simulink model "ACC"  (R2020a)
settings: Solver=FixedStepAuto  StartTime=0.0  StopTime=200  RelTol=1e-3  EnableMultiTasking=on
undefined symbols (not defined in the file): gray
libraries: embdlinuxlib x5, simulink x2, raspberrypiBasiclib x2, dspmtrx3 x1, visionanalysis x1, fuzblock x1, visiongeotforms x1, visiontextngfix x1
settings Model: SimulationMode=external  Creator=Administrator  LastModifiedBy=zhengliang
settings SolverCC: PositivePriorityOrder=on  AutoInsertRateTranBlk=on
settings DataIOCC: ReturnWorkspaceOutputs=off
settings OptimizationCC: EnhancedBackFolding=on  PassReuseOutputArgsAs=Individual arguments  MaxStackSize=64  OptimizeBlockOrder=speed  DifferentSizesBufferReuse=on  OptimizationCustomize=off  EfficientTunableParamExpr=on
settings DebuggingCC: ParameterTunabilityLossMsg=error  ArithmeticOperatorsInVariantConditions=warning
settings HardwareCC: ProdBitPerPointer=32  ProdBitPerSizeT=32  ProdBitPerPtrDiffT=32  ProdLargestAtomicInteger=Long  ProdLargestAtomicFloat=Double  ProdWordSize=32  ProdHWDeviceType=ARM Compatible->ARM Cortex
settings SFSimCC: MATLABDynamicMemAlloc=off  CustomCodeUndefinedFunction=UseInterfaceOnly
settings RTWCC: SystemTargetFile=ert.tlc  HardwareBoard=Raspberry Pi  TemplateMakefile=ert_default_tmf  GenerateReport=on  Toolchain=GNU GCC Raspberry Pi  BuildConfiguration=Faster Runs  IncludeHyperlinkInReport=on  LaunchReport=on  GenerateTraceInfo=on  GenerateTraceReport=on  GenerateTraceReportSl=on  GenerateTraceReportSf=on  GenerateTraceReportEml=on
settings CodeAppCC: ForceParamTrailComments=on  IgnoreCustomStorageClasses=off  OperatorAnnotations=on  SimulinkDataObjDesc=on  SFDataObjDesc=on  InsertBlockDesc=on
settings ERTTargetCC: SupportContinuousTime=on  SupportVariableSizeSignals=on

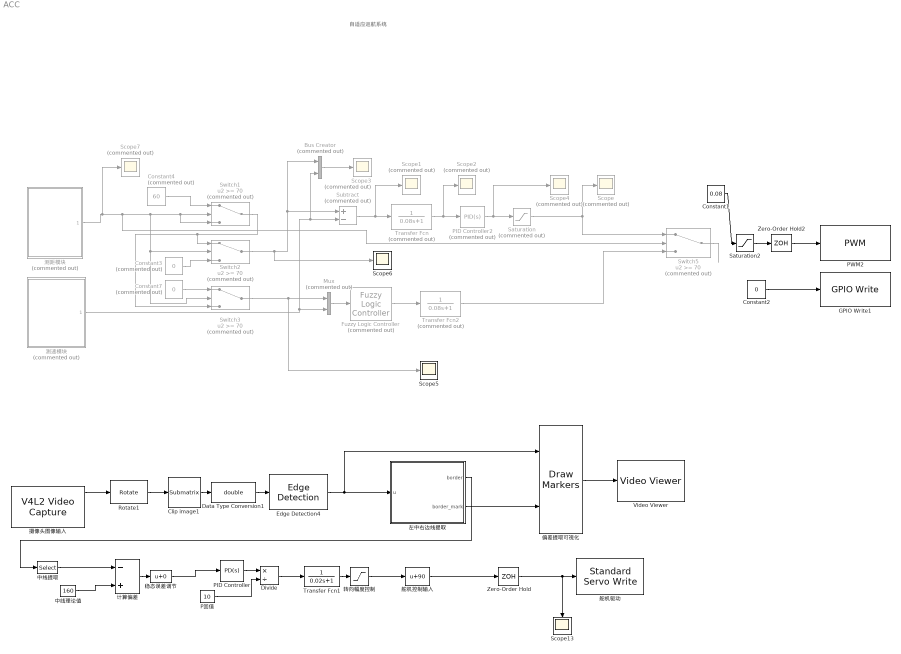
== system ACC ==
  note: 自适应巡航系统
  Bus Creator : BusCreator  Commented=on  Inputs=2
  Clip image1 : dspmtrx3/Submatrix  RowSpan=Range of rows  RowStartMode=Index  RowStartIndex=100  RowEndMode=Index  RowEndIndex=200  ColSpan=All columns  ColStartMode=First  ColStartIndex=1  ColEndMode=Last  ColEndIndex=1
  Constant1 : Constant  Value=0.08
  Constant2 : Constant  Value=0
  Constant3 : Constant  Commented=on  Value=0
  Constant4 : Constant  Commented=on  Value=60
  Constant7 : Constant  Commented=on  Value=0
  Data Type Conversion1 : DataTypeConversion  OutDataTypeStr=double
  Divide : Product  Inputs=*/
  Edge Detection4 : visionanalysis/Edge Detection  method=Sobel  outputType=Binary image  userDefinedThreshold=on  thresholdSource=Specify via dialog  threshold=22  thresholdTuning=1  edgeThinning=on  threshold_canny=[0.25 0.60]  autoPercent=90  sigma=1  roundingMode=Floor  overflowMode=off  prodOutputMode=Binary point scaling  prodOutputWordLength=32  prodOutputFracLength=8
      settings: SourceProductBaseCode=VP
  Fuzzy Logic Controller : fuzblock/Fuzzy Logic  Controller  Commented=on  FIS='tipper.fis'  OutputSampleNumber=101  DataType=double  FuzzifiedInputs=off  RuleFiringStrengths=off  RuleOutputs=off  AggregatedOutputs=off  SimulateUsing=Interpreted execution  OutOfRangeInputValueMessage=warning  NoRuleFiredMessage=warning  EmptyOutputFuzzySetMessage=warning
  GPIO Write1 : embdlinuxlib/GPIO Write  board=Pi 3 Model B+  gpio=27  direction=Output  blockPlatform=Raspberry Pi
      settings: SourceProductBaseCode=SC_BEAGLEBONE_BLUE,RASPPI
  Mux : Mux  Commented=on  Inputs=2
  PID Controller : simulink/Continuous/PID Controller  Controller=PD  Form=Parallel  TimeDomain=Continuous-time  UseExternalTs=off  SampleTime=-1  IntegratorMethod=Forward Euler  FilterMethod=Forward Euler  ControllerParametersSource=internal  P=15  I=0.001  D=0.8  UseFilter=on  N=3  TunerSelectOption=Transfer Function Based (PID Tuner App)  InitialConditionSource=internal  InitialConditionForIntegrator=0  InitialConditionForFilter=0  DifferentiatorICPrevScaledInput=0  ExternalReset=none  TrackingMode=off  Kt=1  LimitOutput=off  UpperSaturationLimit=inf  LowerSaturationLimit=-inf  LinearizeAsGain=on  AntiWindupMode=none  Kb=1  POutMin=[]  POutMax=[]  IOutMin=[]  IOutMax=[]  DOutMin=[]  DOutMax=[]  NOutMin=[]  NOutMax=[]  SumOutMin=[]  SumOutMax=[]  SaturationOutMin=[]  SaturationOutMax=[]  PParamMin=[]  PParamMax=[]  IParamMin=[]  IParamMax=[]  DParamMin=[]  DParamMax=[]  NParamMin=[]  NParamMax=[]  KbParamMin=[]  KbParamMax=[]  KtParamMin=[]  KtParamMax=[]  KbOutMin=[]  KbOutMax=[]  KtOutMin=[]  KtOutMax=[]  IntegratorOutMin=[]  IntegratorOutMax=[]  FilterOutMin=[]  FilterOutMax=[]  SumI1OutMin=[]  SumI1OutMax=[]  SumI2OutMin=[]  SumI2OutMax=[]  SumI3OutMin=[]  SumI3OutMax=[]  SumI4OutMin=[]  SumI4OutMax=[]  SumDOutMin=[]  SumDOutMax=[]  DifferentiatorOutMin=[]  DifferentiatorOutMax=[]  FilterDiffOutCoefMin=[]  FilterDiffOutCoefMax=[]  ReciprocalOutMin=[]  ReciprocalOutMax=[]  SumDenOutMin=[]  SumDenOutMax=[]  SumNumOutMin=[]  SumNumOutMax=[]  DivideOutMin=[]  DivideOutMax=[]  UdiffTsProdOutMin=[]  UdiffTsProdOutMax=[]  NTsProdOutMin=[]  NTsProdOutMax=[]  UintegralTsProdOutMin=[]  UintegralTsProdOutMax=[]  UngainTsProdOutMin=[]  UngainTsProdOutMax=[]  IntegratorContinuousStateAttributes=''  IntegratorStateMustResolveToSignalObject=off  IntegratorRTWStateStorageClass=Auto  FilterContinuousStateAttributes=''  FilterStateMustResolveToSignalObject=off  FilterRTWStateStorageClass=Auto  ParallelPVariant=InternalParameters  IdealPVariant=Disabled  IVariant=Disabled  DVariant=InternalParameters  IntegratorVariant=Disabled  SatVariant=Disabled  AWVariant=Disabled  PCopyVariant=Disabled  TRVariant=Disabled  FdbkBlocksVariant=Forward  IdealPFdbkVariant=Disabled  SatFdbkVariant=Disabled  DerivativeFilterVariant=ContFilter  NVariant=InternalParameters  NCopyVariant=Disabled  FilterICVariant=InternalICsFilter  IntegratorICVariant=Disabled  ExternalResetVariant=Disabled  TRSumVariant=Passthrough  SumFdbkVariant=Disabled  SumVariant=Sum_PD  TsampFilterVariant=InternalTs  TsampNgainVariant=Passthrough  TsampIntegralVariant=Disabled_SignalSpec
  PID Controller2 : simulink/Continuous/PID Controller  Commented=on  Controller=PID  Form=Parallel  TimeDomain=Continuous-time  UseExternalTs=off  SampleTime=-1  IntegratorMethod=Forward Euler  FilterMethod=Forward Euler  ControllerParametersSource=internal  P=0.001  I=0.00005  D=0  UseFilter=on  N=100  TunerSelectOption=Transfer Function Based (PID Tuner App)  InitialConditionSource=internal  InitialConditionForIntegrator=0  InitialConditionForFilter=0  DifferentiatorICPrevScaledInput=0  ExternalReset=none  TrackingMode=off  Kt=1  LimitOutput=off  UpperSaturationLimit=inf  LowerSaturationLimit=-inf  LinearizeAsGain=on  AntiWindupMode=none  Kb=1  POutMin=[]  POutMax=[]  IOutMin=[]  IOutMax=[]  DOutMin=[]  DOutMax=[]  NOutMin=[]  NOutMax=[]  SumOutMin=[]  SumOutMax=[]  SaturationOutMin=[]  SaturationOutMax=[]  PParamMin=[]  PParamMax=[]  IParamMin=[]  IParamMax=[]  DParamMin=[]  DParamMax=[]  NParamMin=[]  NParamMax=[]  KbParamMin=[]  KbParamMax=[]  KtParamMin=[]  KtParamMax=[]  KbOutMin=[]  KbOutMax=[]  KtOutMin=[]  KtOutMax=[]  IntegratorOutMin=[]  IntegratorOutMax=[]  FilterOutMin=[]  FilterOutMax=[]  SumI1OutMin=[]  SumI1OutMax=[]  SumI2OutMin=[]  SumI2OutMax=[]  SumI3OutMin=[]  SumI3OutMax=[]  SumI4OutMin=[]  SumI4OutMax=[]  SumDOutMin=[]  SumDOutMax=[]  DifferentiatorOutMin=[]  DifferentiatorOutMax=[]  FilterDiffOutCoefMin=[]  FilterDiffOutCoefMax=[]  ReciprocalOutMin=[]  ReciprocalOutMax=[]  SumDenOutMin=[]  SumDenOutMax=[]  SumNumOutMin=[]  SumNumOutMax=[]  DivideOutMin=[]  DivideOutMax=[]  UdiffTsProdOutMin=[]  UdiffTsProdOutMax=[]  NTsProdOutMin=[]  NTsProdOutMax=[]  UintegralTsProdOutMin=[]  UintegralTsProdOutMax=[]  UngainTsProdOutMin=[]  UngainTsProdOutMax=[]  IntegratorContinuousStateAttributes=''  IntegratorStateMustResolveToSignalObject=off  IntegratorRTWStateStorageClass=Auto  FilterContinuousStateAttributes=''  FilterStateMustResolveToSignalObject=off  FilterRTWStateStorageClass=Auto  ParallelPVariant=InternalParameters  IdealPVariant=Disabled  IVariant=InternalParameters  DVariant=InternalParameters  IntegratorVariant=Continuous  SatVariant=Disabled  AWVariant=Passthrough  PCopyVariant=Disabled  TRVariant=Disabled  FdbkBlocksVariant=Forward  IdealPFdbkVariant=Disabled  SatFdbkVariant=Disabled  DerivativeFilterVariant=ContFilter  NVariant=InternalParameters  NCopyVariant=Disabled  FilterICVariant=InternalICsFilter  IntegratorICVariant=InternalICs  ExternalResetVariant=Disabled  TRSumVariant=Passthrough  SumFdbkVariant=Disabled  SumVariant=Sum_PID  TsampFilterVariant=InternalTs  TsampNgainVariant=Passthrough  TsampIntegralVariant=Passthrough
  PWM2 : raspberrypiBasiclib/PWM  board=Pi 3 Model B+  Pin_=17  Frequency=8000  blockPlatform=Raspberry Pi
      settings: SourceProductBaseCode=RASPPI
  P回值 : Constant  Value=10
  Rotate1 : visiongeotforms/Rotate  outSizeR=Expanded to fit rotated input image  src_angle=Specify via dialog  unit_angle=Degrees  angle=-pi/2  maxAngle=pi  dispImage=Top-left corner  method=Table lookup  fillVal=0  interpMethod=Bilinear  roundingMode=Nearest  overflowMode=on  prodOutputMode=Binary point scaling  prodOutputWordLength=32  prodOutputFracLength=10
      settings: LockScale=on
  Saturation : Saturate  Commented=on  UpperLimit=0.071  LowerLimit=0.07
  Saturation2 : Saturate  UpperLimit=0.2  LowerLimit=0
  Scope{,1..4,7} (6 alike) : Scope  Commented=on
  Scope13 : Scope
  Scope5 : Scope
  Scope6 : Scope
  Subtract : Sum  Commented=on  Inputs=+-
  Switch{1..3,5} (4 alike) : Switch  Commented=on  Threshold=70
  Transfer Fcn : TransferFcn  Commented=on  Denominator=[0.08 1]
  Transfer Fcn1 : TransferFcn  Denominator=[0.02 1]
  Transfer Fcn2 : TransferFcn  Commented=on  Denominator=[0.08 1]
  Video Viewer : VideoViewer  colormapValue=gray(256)  FigPos=[253 673 766 511]
  Zero-Order Hold : ZeroOrderHold  SampleTime=0.05
  Zero-Order Hold2 : ZeroOrderHold  SampleTime=0.05
  中线提取 : Selector  NumberOfDimensions=2  InputPortWidth=3  IndexOptions=Index vector (dialog),Index vector (dialog)  Indices=[2],2  OutputSizes=1,1
  中线理论值 : Constant  Value=160
  偏差提取可视化 : visiontextngfix/Draw Markers  shape=Circle  size=3  fill=off  fillClrSource=Specify via dialog  display=White  intensity=200  color=[200 255 100]  opacity=0.6  viewport=Entire image  antialiasing=off  inType=Obsolete  imagePorts=One multidimensional signal  roundingMode=Floor  overflowMode=off  memoryMode=Specify word length  memoryWordLength=16  memoryFracLength=15  prodOutputMode=Binary point scaling  prodOutputWordLength=32  prodOutputFracLength=14
      settings: SourceProductBaseCode=VP
  左中右边线提取 : MATLAB Function  TreatAsAtomicUnit=on
  摄像头图像输入 : embdlinuxlib/V4L2 Video Capture  m_devName='/dev/video0'  roi=[0, 0, 640, 480]  imSizeSelection=320x240  imSize=[640, 480]  pixelFormat=RGB  pixelOrder=Planar  sampleTime=1/50  simOutput=Colorbars  blockPlatform=Raspberry Pi
      settings: SourceProductBaseCode=SC_BEAGLEBONE_BLUE,RASPPI
  "测距模块 " : Subsystem  Commented=on
  "测速模块 " : Subsystem  Commented=on
  稳态误差调节 : Bias
  舵机控制输入 : Bias  Bias=90
  舵机驱动 : raspberrypiBasiclib/Standard Servo Write  board=Pi 3 Model B+  Pin_=21  MinPulseDuration=0.96e-3  MaxPulseDuration=1.96e-3  blockPlatform=Raspberry Pi
      settings: SourceProductBaseCode=RASPPI
  计算偏差 : Sum  Inputs=-+
  转向幅度控制 : Saturate  UpperLimit=85  LowerLimit=-85
  wires:
  P回值/1 -> Divide/2
  Transfer Fcn1/1 -> 转向幅度控制/1
  Divide/1 -> Transfer Fcn1/1
  左中右边线提取/1(border) -> 中线提取/1
  Zero-Order Hold/1 -> 舵机驱动/1, Scope13/1
  舵机控制输入/1 -> Zero-Order Hold/1
  中线理论值/1 -> 计算偏差/2
  左中右边线提取/2(border_mark) -> 偏差提取可视化/2
  Clip image1/1 -> Data Type Conversion1/1
  Rotate1/1 -> Clip image1/1
  转向幅度控制/1 -> 舵机控制输入/1
  偏差提取可视化/1 -> Video Viewer/1
  稳态误差调节/1 -> PID Controller/1
  PID Controller/1 -> Divide/1
  Data Type Conversion1/1 -> Edge Detection4/1
  中线提取/1 -> 计算偏差/1
  摄像头图像输入/1 -> Rotate1/1
  计算偏差/1 -> 稳态误差调节/1
  Edge Detection4/1 -> 偏差提取可视化/1, 左中右边线提取/1(u)
  "测距模块 "/1(" ") -> Scope7/1, Switch5/2, Switch3/2, Switch2/2, Switch1/2, Switch1/3
  Constant2/1 -> GPIO Write1/1
  Saturation2/1 -> Zero-Order Hold2/1
  Zero-Order Hold2/1 -> PWM2/1
  Constant4/1 -> Switch1/1
  Saturation/1 -> Switch5/1, Scope/1
  Subtract/1 -> Scope1/1, Transfer Fcn/1
  PID Controller2/1 -> Saturation/1, Scope4/1
  Bus Creator/1 -> Scope3/1
  Transfer Fcn/1 -> PID Controller2/1, Scope2/1
  Switch1/1 -> Switch2/1, Switch3/3
  Constant3/1 -> Switch2/3
  Switch2/1 -> Scope6/1, Subtract/1, Bus Creator/1
  Constant7/1 -> Switch3/1
  Fuzzy Logic Controller/1 -> Transfer Fcn2/1
  "测速模块 "/1(" ") -> Mux/2, Subtract/2, Bus Creator/2
  Switch3/1 -> Scope5/1, Mux/1
  Mux/1 -> Fuzzy Logic Controller/1
  Transfer Fcn2/1 -> Switch5/3
  Switch5/1 -> ?
  Constant1/1 -> Saturation2/1

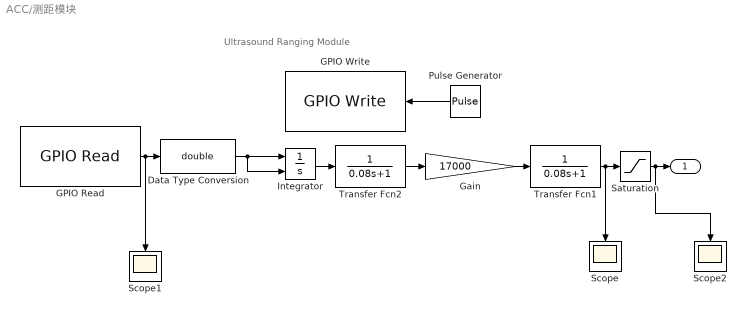
== system ACC/测距模块  ==
  note: Ultrasound Ranging Module
  Data Type Conversion : DataTypeConversion  OutDataTypeStr=double
  GPIO Read : embdlinuxlib/GPIO Read  board=Pi 3 Model B+  gpio=24  internalResistor=Off  sampleTime=inf  direction=Input  blockPlatform=Raspberry Pi
      settings: SourceProductBaseCode=SC_BEAGLEBONE_BLUE,RASPPI
  GPIO Write : embdlinuxlib/GPIO Write  board=Pi 3 Model B+  gpio=23  direction=Output  blockPlatform=Raspberry Pi
      settings: SourceProductBaseCode=SC_BEAGLEBONE_BLUE,RASPPI
  Gain : Gain  Gain=17000
  Integrator : Integrator  ExternalReset=rising
  Pulse Generator : DiscretePulseGenerator  PulseType=Time based  Period=0.1  PulseWidth=50
  Saturation : Saturate  UpperLimit=100  LowerLimit=0
  Scope : Scope
  Scope1 : Scope
  Scope2 : Scope
  Transfer Fcn1 : TransferFcn  Denominator=[0.08 1]
  Transfer Fcn2 : TransferFcn  Denominator=[0.08 1]
  " " : Outport  VectorParamsAs1DForOutWhenUnconnected=off
  wires:
  Data Type Conversion/1 -> Integrator/2, Integrator/1
  Pulse Generator/1 -> GPIO Write/1
  GPIO Read/1 -> Scope1/1, Data Type Conversion/1
  Gain/1 -> Transfer Fcn1/1
  Integrator/1 -> Transfer Fcn2/1
  Transfer Fcn1/1 -> Scope/1, Saturation/1
  Transfer Fcn2/1 -> Gain/1
  Saturation/1 -> Scope2/1, " "/1

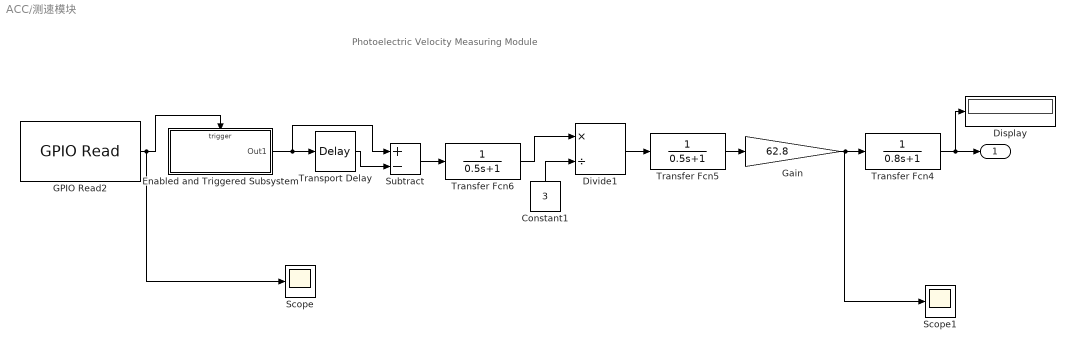
== system ACC/测速模块  ==
  note: Photoelectric Velocity Measuring Module
  Constant1 : Constant  Value=3
  Display : Display
  Divide1 : Product  Inputs=*/
  Enabled and Triggered Subsystem : Subsystem  TreatAsAtomicUnit=on
  GPIO Read2 : embdlinuxlib/GPIO Read  board=Pi 3 Model B+  gpio=21  internalResistor=Off  sampleTime=0.01  direction=Input  blockPlatform=Raspberry Pi
      settings: SourceProductBaseCode=SC_BEAGLEBONE_BLUE,RASPPI
  Gain : Gain  Gain=62.8
  Scope : Scope
  Scope1 : Scope
  Subtract : Sum  Inputs=+-
  Transfer Fcn4 : TransferFcn  Denominator=[0.8 1]
  Transfer Fcn5 : TransferFcn  Denominator=[0.5 1]
  Transfer Fcn6 : TransferFcn  Denominator=[0.5 1]
  Transport Delay : TransportDelay  DelayTime=0.5
  " " : Outport  VectorParamsAs1DForOutWhenUnconnected=off
  wires:
  Constant1/1 -> Divide1/2
  Enabled and Triggered Subsystem/1(Out1) -> Transport Delay/1, Subtract/1
  Transfer Fcn6/1 -> Divide1/1
  Transport Delay/1 -> Subtract/2
  Transfer Fcn5/1 -> Gain/1
  Divide1/1 -> Transfer Fcn5/1
  Transfer Fcn4/1 -> " "/1, Display/1
  Gain/1 -> Scope1/1, Transfer Fcn4/1
  Subtract/1 -> Transfer Fcn6/1
  GPIO Read2/1 -> Scope/1, Enabled and Triggered Subsystem/Trigger

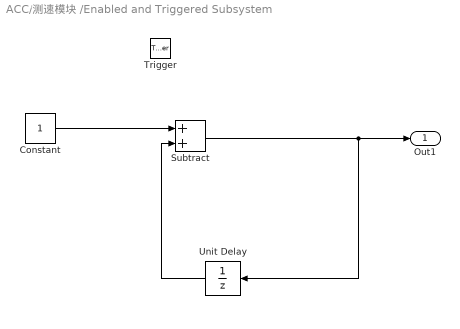
== system ACC/测速模块 /Enabled and Triggered Subsystem ==
  Trigger : TriggerPort  TriggerType=falling  VariantControl=Variant
  Constant : Constant
  Subtract : Sum
  Unit Delay : UnitDelay  SampleTime=-1  HasFrameUpgradeWarning=on
  Out1 : Outport  VectorParamsAs1DForOutWhenUnconnected=off
  wires:
  Constant/1 -> Subtract/1
  Subtract/1 -> Unit Delay/1, Out1/1
  Unit Delay/1 -> Subtract/2

== matlab function ACC/左中右边线提取 ==
  data: u input; border output; border_mark output
function [border,border_mark]= fcn(u)
scan_line=[100 75 50 25];
scan_lines=length(scan_line);
border=zeros(scan_lines,3);
[~,x_max]=size(u);
x_max_2 = x_max/2;
for i=1:scan_lines
    border(i,3)= x_max;
    border(i,2)= x_max_2;
end
mid = x_max_2;
%start to scan the border
for y=1:scan_lines
    for x_left=1:mid
        if u(scan_line(y),mid-x_left+1)==1
           border(y,1)=x_max_2-x_left;
           break
        end
    end
    for x_right=1:(x_max-mid)
        if u(scan_line(y),mid+x_right-1)==1
           border(y,3)=x_max_2+x_right;
           break
        end
    end
    border(y,2)=(border(y,1)+border(y,3))/2;
    mid = border(y,2);
end
%output the border in video
border_mark =int16(zeros(scan_lines*3,2));
for y=1:scan_lines*3
    border_mark(y,2)=scan_line(fix(y/3.1+1));
    border_mark(y,1)=border(fix(y/3.1+1),rem(y+2,3)+1);
end
